simulink model "Inverted Pendulum stabilization_unstable_equilibrium"  (R2022b)
settings: Solver=VariableStepAuto  StartTime=0  StopTime=50  RelTol=1e-3
libraries: simulink x5, slpidlib x3
settings Model: Creator=Shaan Sapru  LastModifiedBy=Shaan Sapru
settings DataIOCC: SaveFormat=StructureWithTime
settings OptimizationCC: BlockReduction=off  BufferReuse=off
settings DebuggingCC: AlgebraicLoopMsg=none
settings ExplorerConfigSet: SimMechanicsOpenEditorOnUpdate=off

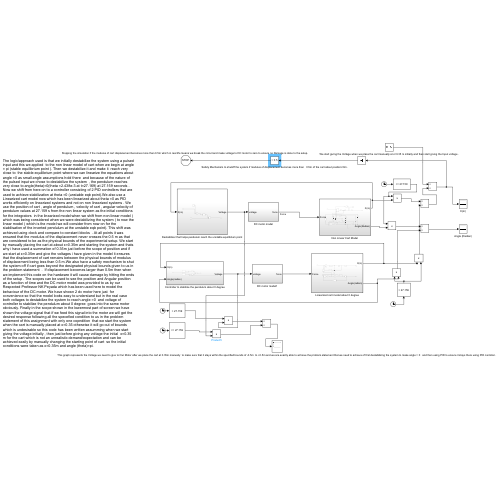
[thumbnail: Simulink's stored preview of the top-level diagram]
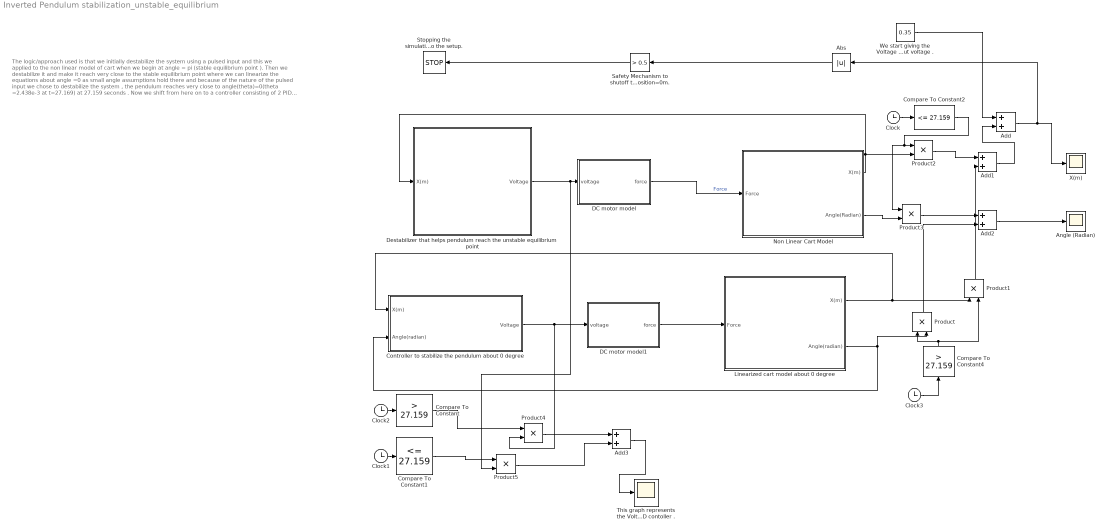
== system Inverted Pendulum stabilization_unstable_equilibrium ==
  note: The logic/approach used is that we initially destabilize the system using a pulsed input and this we applied to the non linear model of cart when we begin at angle = pi (stable equilibrium point ). Then we destabilize it and make it reach very close to the stable equilibrium point where we can linearize the equations about angle =0 as small angle assumptions hold there and because of the nature of the pulsed input we chose to destabilize the system , the pendulum reaches very close to angle(theta)=0(theta =2.438e-3 at t=27.169) at 27.159 seconds . Now we shift from here on to a controller consisting of 2 PID controllers that are used to achieve stabilization at theta =0 (unstable eqb point).We also use a Linearized cart model now which has been linearized about theta =0 as PID works efficiently on linearized systems and not on non linearized systems . We use the position of cart , angle of pendulum , velocity of cart , angular velocity of pendulum values at 27.159 s from the non linear system as the initial conditions for the integrators in the linearized model when we shift from non linear model ( which was being considered when we were destabilizing the system ) to now the linear model ( which is the model we will consider from now on for the stabilisation of the inverted pendulum at the unstable eqb point). This shift was achieved using clock and compare to constant blocks . At all points it was ensured that the modulus of the displacement never crosses the 0.5 m as that are considered to be as the physical bounds of the experimental setup. We start by manually placing the cart at about x=0.35m and starting the system and thats why i have used a summation of 0.35m just before the scope of position and if we start at x=0.35m and give the voltages i have given in the model it ensures that the displacement of cart remains between the physical bounds of modulus of displacement being less than 0.5 m.We also have a safety mechanism to shut the system off if cart goes beyond the designated physical bounds given to us in the problem statement . If displacement becomes larger than 0.5m then when we implement this code on the hardware it will cause damage by hitting the ends of the setup . The scopes can be used to see the position and Angular position as a function of time and the DC motor model was provided to us by our Respected Professor NK Peyada which has been used here to model the behaviour of the DC motor. We have shown 2 dc motor here just for convenience so that the model looks easy to understand but in the real case both voltages to destabilize the system to reach angle =0 and voltage of controller to stabilize the pendulum about 0 degree goes into the same motor obviously. Finally in the scope shown in the lowermost part of screen we have shown the voltage signal that if we feed this signal into the motor we will get the desired response following all the specefied condition to us in the problem statement of this assignment with only one copndition that we start the system when the cart is manually placed at x=0.35 otherwise it will go out of bounds which is undesirable so this code has been written assumming when we start giving the voltage initially , then just before giving any voltage the initial x=0.35 m for the cart which is not an unrealistic demand/expectation and can be achieved easily by manually changing the starting point of cart so the initial conditions were taken as x=0.35m and angle (theta)=pi.
  Abs : Abs  SaturateOnIntegerOverflow=off
  Add{,1..3} (4 alike) : Sum
  Angle (Radian) : Scope
  Clock{,1..3} (4 alike) : Clock
  Compare To Constant : simulink/Logic and Bit Operations/Compare To Constant  relop=>  const=27.159  OutDataTypeStr=boolean
  Compare To Constant1 : simulink/Logic and Bit Operations/Compare To Constant  relop=<=  const=27.159  OutDataTypeStr=boolean
  Compare To Constant2 : simulink/Logic and Bit Operations/Compare To Constant  relop=<=  const=27.159  OutDataTypeStr=boolean
  Compare To Constant4 : simulink/Logic and Bit Operations/Compare To Constant  relop=>  const=27.159  OutDataTypeStr=boolean
  Controller to stabilize the pendulum about 0 degree : Subsystem
  DC motor model : Subsystem
  DC motor model1 : Subsystem
  Destabilizer that helps pendulum reach the unstable equilibrium point : Subsystem
  Linearized cart model about 0 degree : Subsystem
  "Non Linear Cart Model " : Subsystem
  Product{,1..5} (6 alike) : Product
  Safety Mechanism to shutoff the system if modulus of displacement becomes more than   0.5m of the cart about position=0m. : simulink/Logic and Bit Operations/Compare To Constant  relop=>  const=0.5  OutDataTypeStr=boolean
  "Stopping the simulation if the modulus of cart displacement becomes more than 0.5m which in real life means we break the circuit and make voltage to DC motor to zero to ensure no Damage is done to the setup.  " : Stop
  "This graph represents the Voltage we need to give to Our Motor after we place the cart at 0.35m manually  to make sure that it stays within the specified bounds of -0.5m  to +0.5m and we are exactly able to achieve the problem statement that we need to achieve of first destabilizing the system to make angle = 0   and then using PID to ensure it stays there using PID contoller . " : Scope
  We start giving the Voltage when we place the cart manually at x=0.35 m initially and then start giving the Input voltage . : Constant  Value=0.35
  X(m) : Scope
  wires:
  DC motor model/1(force) -> "Non Linear Cart Model "/1(Force)  "Force"
  "Non Linear Cart Model "/1(X(m)) -> Product2/2, Destabilizer that helps pendulum reach the unstable equilibrium point/1(X(m))
  Destabilizer that helps pendulum reach the unstable equilibrium point/1(Voltage) -> Product5/2, DC motor model/1(voltage)
  DC motor model1/1(force) -> Linearized cart model about 0 degree/1(Force)
  Linearized cart model about 0 degree/1(X(m)) -> Controller to stabilize the pendulum about 0 degree/1(X(m)), Product1/1
  Linearized cart model about 0 degree/2(Angle(radian)) -> Controller to stabilize the pendulum about 0 degree/2(Angle(radian)), Product/2
  Add2/1 -> Angle (Radian)/1
  Add1/1 -> Add/2
  Product/1 -> Add2/2
  Product1/1 -> Add1/2
  Controller to stabilize the pendulum about 0 degree/1(Voltage) -> Product4/2, DC motor model1/1(voltage)
  Clock3/1 -> Compare To Constant4/1
  Compare To Constant4/1 -> Product/1, Product1/2
  Clock/1 -> Compare To Constant2/1
  Compare To Constant2/1 -> Product3/1, Product2/1
  Product2/1 -> Add1/1
  "Non Linear Cart Model "/2(Angle(Radian)) -> Product3/2
  Product3/1 -> Add2/1
  Safety Mechanism to shutoff the system if modulus of displacement becomes more than   0.5m of the cart about position=0m./1 -> "Stopping the simulation if the modulus of cart displacement becomes more than 0.5m which in real life means we break the circuit and make voltage to DC motor to zero to ensure no Damage is done to the setup.  "/1
  Abs/1 -> Safety Mechanism to shutoff the system if modulus of displacement becomes more than   0.5m of the cart about position=0m./1
  We start giving the Voltage when we place the cart manually at x=0.35 m initially and then start giving the Input voltage ./1 -> Add/1
  Add/1 -> Abs/1, X(m)/1
  Add3/1 -> "This graph represents the Voltage we need to give to Our Motor after we place the cart at 0.35m manually  to make sure that it stays within the specified bounds of -0.5m  to +0.5m and we are exactly able to achieve the problem statement that we need to achieve of first destabilizing the system to make angle = 0   and then using PID to ensure it stays there using PID contoller . "/1
  Compare To Constant/1 -> Product4/1
  Compare To Constant1/1 -> Product5/1
  Clock1/1 -> Compare To Constant1/1
  Product5/1 -> Add3/2
  Clock2/1 -> Compare To Constant/1
  Product4/1 -> Add3/1

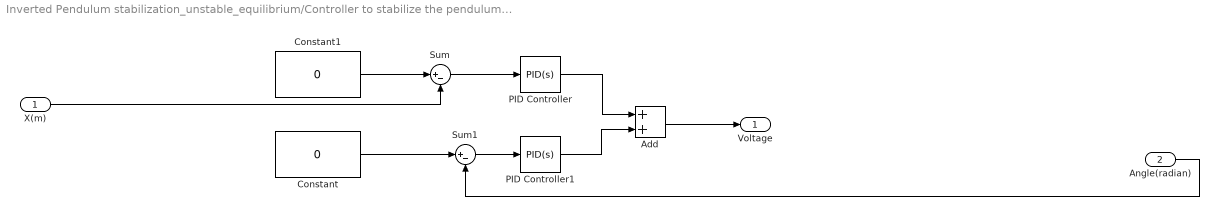
== system Inverted Pendulum stabilization_unstable_equilibrium/Controller to stabilize the pendulum about 0 degree ==
  X(m) : Inport
  Angle(radian) : Inport  Port=2
  Add : Sum
  Constant : Constant  Value=0
  Constant1 : Constant  Value=0
  PID Controller : slpidlib/PID Controller  Controller=PID  Form=Parallel  TimeDomain=Continuous-time  UseExternalTs=off  SampleTime=-1  IntegratorMethod=Forward Euler  FilterMethod=Forward Euler  ControllerParametersSource=internal  P=832.0243  I=93.876  UseKiTs=off  D=-197.943  N=4.2033  UseFilter=on  TunerSelectOption=Transfer Function Based (PID Tuner App)  InitialConditionSource=internal  InitialConditionForIntegrator=0  InitialConditionForFilter=0  DifferentiatorICPrevScaledInput=0  ExternalReset=none  TrackingMode=off  Kt=1  LimitOutput=off  SatLimitsSource=internal  UpperSaturationLimit=inf  LowerSaturationLimit=-inf  LinearizeAsGain=on  AntiWindupMode=none  Kb=1  LimitIntegrator=off  UpperIntegratorSaturationLimit=inf  LowerIntegratorSaturationLimit=-inf  POutMin=[]  POutMax=[]  IOutMin=[]  IOutMax=[]  DOutMin=[]  DOutMax=[]  NOutMin=[]  NOutMax=[]  SumOutMin=[]  SumOutMax=[]  SaturationOutMin=[]  SaturationOutMax=[]  PParamMin=[]  PParamMax=[]  IParamMin=[]  IParamMax=[]  DParamMin=[]  DParamMax=[]  NParamMin=[]  NParamMax=[]  KbParamMin=[]  KbParamMax=[]  KtParamMin=[]  KtParamMax=[]  KbOutMin=[]  KbOutMax=[]  KtOutMin=[]  KtOutMax=[]  IntegratorOutMin=[]  IntegratorOutMax=[]  FilterOutMin=[]  FilterOutMax=[]  SumI1OutMin=[]  SumI1OutMax=[]  SumI2OutMin=[]  SumI2OutMax=[]  SumI3OutMin=[]  SumI3OutMax=[]  SumI4OutMin=[]  SumI4OutMax=[]  SumDOutMin=[]  SumDOutMax=[]  DifferentiatorOutMin=[]  DifferentiatorOutMax=[]  FilterDiffOutCoefMin=[]  FilterDiffOutCoefMax=[]  ReciprocalOutMin=[]  ReciprocalOutMax=[]  SumDenOutMin=[]  SumDenOutMax=[]  SumNumOutMin=[]  SumNumOutMax=[]  DivideOutMin=[]  DivideOutMax=[]  UdiffTsProdOutMin=[]  UdiffTsProdOutMax=[]  NTsProdOutMin=[]  NTsProdOutMax=[]  UintegralTsProdOutMin=[]  UintegralTsProdOutMax=[]  UngainTsProdOutMin=[]  UngainTsProdOutMax=[]  ClampingZeroOutDataTypeStr=Inherit: Inherit via back propagation  ClampingZeroOutMin=[]  ClampingZeroOutMax=[]  FilterDenConstantOutDataTypeStr=Inherit: Inherit via back propagation  FilterDenConstantOutMin=[]  FilterDenConstantOutMax=[]  PCopyOutDataTypeStr=Inherit: Inherit via back propagation  PCopyOutMin=[]  PCopyOutMax=[]  NCopyOutDataTypeStr=Inherit: Inherit via back propagation  NCopyOutMin=[]  NCopyOutMax=[]  IntegratorContinuousStateAttributes=''  IntegratorStateMustResolveToSignalObject=off  IntegratorRTWStateStorageClass=Auto  FilterContinuousStateAttributes=''  FilterStateMustResolveToSignalObject=off  FilterRTWStateStorageClass=Auto  ParallelPVariant=InternalParameters  IdealPVariant=Disabled  IVariant=InternalParameters  DVariant=InternalParameters  IntegratorVariant=Continuous  SatVariant=Disabled  AWVariant=Passthrough  PCopyVariant=Disabled  TRVariant=Disabled  FdbkBlocksVariant=Forward  IdealPFdbkVariant=Disabled  SatFdbkVariant=Disabled  DerivativeFilterVariant=ContFilter  NVariant=InternalParameters  NCopyVariant=Disabled  FilterICVariant=InternalICsFilter  IntegratorICVariant=InternalICs  ExternalResetVariant=Disabled  TRSumVariant=Passthrough  SumFdbkVariant=Disabled  SumVariant=Sum_PID  TsampFilterVariant=InternalTs  TsampNgainVariant=Passthrough  TsampIntegralVariant=Passthrough  ExternalSaturationOutDataTypeStr=Inherit: Same as second input
  PID Controller1 : slpidlib/PID Controller  Controller=PID  Form=Parallel  TimeDomain=Continuous-time  UseExternalTs=off  SampleTime=-1  IntegratorMethod=Forward Euler  FilterMethod=Forward Euler  ControllerParametersSource=internal  P=2215.083  I=8077.564  UseKiTs=off  D=0  N=100  UseFilter=on  TunerSelectOption=Transfer Function Based (PID Tuner App)  InitialConditionSource=internal  InitialConditionForIntegrator=0  InitialConditionForFilter=0  DifferentiatorICPrevScaledInput=0  ExternalReset=none  TrackingMode=off  Kt=1  LimitOutput=off  SatLimitsSource=internal  UpperSaturationLimit=inf  LowerSaturationLimit=-inf  LinearizeAsGain=on  AntiWindupMode=none  Kb=1  LimitIntegrator=off  UpperIntegratorSaturationLimit=inf  LowerIntegratorSaturationLimit=-inf  POutMin=[]  POutMax=[]  IOutMin=[]  IOutMax=[]  DOutMin=[]  DOutMax=[]  NOutMin=[]  NOutMax=[]  SumOutMin=[]  SumOutMax=[]  SaturationOutMin=[]  SaturationOutMax=[]  PParamMin=[]  PParamMax=[]  IParamMin=[]  IParamMax=[]  DParamMin=[]  DParamMax=[]  NParamMin=[]  NParamMax=[]  KbParamMin=[]  KbParamMax=[]  KtParamMin=[]  KtParamMax=[]  KbOutMin=[]  KbOutMax=[]  KtOutMin=[]  KtOutMax=[]  IntegratorOutMin=[]  IntegratorOutMax=[]  FilterOutMin=[]  FilterOutMax=[]  SumI1OutMin=[]  SumI1OutMax=[]  SumI2OutMin=[]  SumI2OutMax=[]  SumI3OutMin=[]  SumI3OutMax=[]  SumI4OutMin=[]  SumI4OutMax=[]  SumDOutMin=[]  SumDOutMax=[]  DifferentiatorOutMin=[]  DifferentiatorOutMax=[]  FilterDiffOutCoefMin=[]  FilterDiffOutCoefMax=[]  ReciprocalOutMin=[]  ReciprocalOutMax=[]  SumDenOutMin=[]  SumDenOutMax=[]  SumNumOutMin=[]  SumNumOutMax=[]  DivideOutMin=[]  DivideOutMax=[]  UdiffTsProdOutMin=[]  UdiffTsProdOutMax=[]  NTsProdOutMin=[]  NTsProdOutMax=[]  UintegralTsProdOutMin=[]  UintegralTsProdOutMax=[]  UngainTsProdOutMin=[]  UngainTsProdOutMax=[]  ClampingZeroOutDataTypeStr=Inherit: Inherit via back propagation  ClampingZeroOutMin=[]  ClampingZeroOutMax=[]  FilterDenConstantOutDataTypeStr=Inherit: Inherit via back propagation  FilterDenConstantOutMin=[]  FilterDenConstantOutMax=[]  PCopyOutDataTypeStr=Inherit: Inherit via back propagation  PCopyOutMin=[]  PCopyOutMax=[]  NCopyOutDataTypeStr=Inherit: Inherit via back propagation  NCopyOutMin=[]  NCopyOutMax=[]  IntegratorContinuousStateAttributes=''  IntegratorStateMustResolveToSignalObject=off  IntegratorRTWStateStorageClass=Auto  FilterContinuousStateAttributes=''  FilterStateMustResolveToSignalObject=off  FilterRTWStateStorageClass=Auto  ParallelPVariant=InternalParameters  IdealPVariant=Disabled  IVariant=InternalParameters  DVariant=InternalParameters  IntegratorVariant=Continuous  SatVariant=Disabled  AWVariant=Passthrough  PCopyVariant=Disabled  TRVariant=Disabled  FdbkBlocksVariant=Forward  IdealPFdbkVariant=Disabled  SatFdbkVariant=Disabled  DerivativeFilterVariant=ContFilter  NVariant=InternalParameters  NCopyVariant=Disabled  FilterICVariant=InternalICsFilter  IntegratorICVariant=InternalICs  ExternalResetVariant=Disabled  TRSumVariant=Passthrough  SumFdbkVariant=Disabled  SumVariant=Sum_PID  TsampFilterVariant=InternalTs  TsampNgainVariant=Passthrough  TsampIntegralVariant=Passthrough  ExternalSaturationOutDataTypeStr=Inherit: Same as second input
  Sum : Sum  Inputs=|+-
  Sum1 : Sum  Inputs=|+-
  Voltage : Outport
  wires:
  Constant1/1 -> Sum/1
  PID Controller1/1 -> Add/2
  Add/1 -> Voltage/1
  Constant/1 -> Sum1/1
  PID Controller/1 -> Add/1
  Sum1/1 -> PID Controller1/1
  X(m)/1 -> Sum/2
  Sum/1 -> PID Controller/1
  Angle(radian)/1 -> Sum1/2

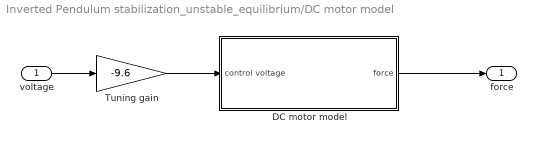
== system Inverted Pendulum stabilization_unstable_equilibrium/DC motor model ==
  voltage : Inport
  DC motor model : Subsystem  mask{J=0.0000140, Kt=0.05, Kb=0.05, d=0.000001, R=2.5, L=0.0025}
      mask prompts: J "Moment of inertia"; Kt "Torque constant"; Kb "Electromotive force constant"; d "Linear approximation of viscous friction"; R "Electrical circuit resistance"; L "Electrical circuit inductance"
      mask Display: disp('DC motor')
  Tuning gain : Gain  Gain=-9.6
  force : Outport
  wires:
  Tuning gain/1 -> DC motor model/1(control voltage)
  voltage/1 -> Tuning gain/1
  DC motor model/1(force) -> force/1

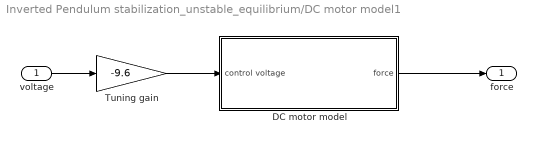
== system Inverted Pendulum stabilization_unstable_equilibrium/DC motor model1 ==
  voltage : Inport
  DC motor model : Subsystem  mask{J=0.0000140, Kt=0.05, Kb=0.05, d=0.000001, R=2.5, L=0.0025}
      mask prompts: J "Moment of inertia"; Kt "Torque constant"; Kb "Electromotive force constant"; d "Linear approximation of viscous friction"; R "Electrical circuit resistance"; L "Electrical circuit inductance"
      mask Display: disp('DC motor')
  Tuning gain : Gain  Gain=-9.6
  force : Outport
  wires:
  Tuning gain/1 -> DC motor model/1(control voltage)
  voltage/1 -> Tuning gain/1
  DC motor model/1(force) -> force/1

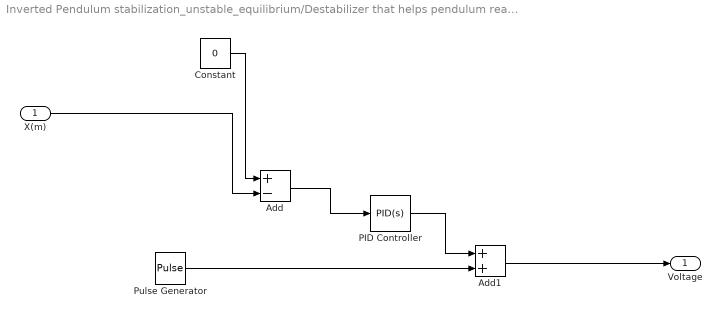
== system Inverted Pendulum stabilization_unstable_equilibrium/Destabilizer that helps pendulum reach the unstable equilibrium point ==
  X(m) : Inport
  Add : Sum  Inputs=+-
  Add1 : Sum
  Constant : Constant  Value=0
  PID Controller : slpidlib/PID Controller  Controller=PID  Form=Parallel  TimeDomain=Continuous-time  UseExternalTs=off  SampleTime=-1  IntegratorMethod=Forward Euler  FilterMethod=Forward Euler  ControllerParametersSource=internal  P=-0.689804794145449  I=-0.0287985752446261  UseKiTs=off  D=-0.351556934511218  N=2.44257175027819  UseFilter=on  TunerSelectOption=Transfer Function Based (PID Tuner App)  InitialConditionSource=internal  InitialConditionForIntegrator=0  InitialConditionForFilter=0  DifferentiatorICPrevScaledInput=0  ExternalReset=none  TrackingMode=off  Kt=1  LimitOutput=off  SatLimitsSource=internal  UpperSaturationLimit=inf  LowerSaturationLimit=-inf  LinearizeAsGain=on  AntiWindupMode=none  Kb=1  LimitIntegrator=off  UpperIntegratorSaturationLimit=inf  LowerIntegratorSaturationLimit=-inf  POutMin=[]  POutMax=[]  IOutMin=[]  IOutMax=[]  DOutMin=[]  DOutMax=[]  NOutMin=[]  NOutMax=[]  SumOutMin=[]  SumOutMax=[]  SaturationOutMin=[]  SaturationOutMax=[]  PParamMin=[]  PParamMax=[]  IParamMin=[]  IParamMax=[]  DParamMin=[]  DParamMax=[]  NParamMin=[]  NParamMax=[]  KbParamMin=[]  KbParamMax=[]  KtParamMin=[]  KtParamMax=[]  KbOutMin=[]  KbOutMax=[]  KtOutMin=[]  KtOutMax=[]  IntegratorOutMin=[]  IntegratorOutMax=[]  FilterOutMin=[]  FilterOutMax=[]  SumI1OutMin=[]  SumI1OutMax=[]  SumI2OutMin=[]  SumI2OutMax=[]  SumI3OutMin=[]  SumI3OutMax=[]  SumI4OutMin=[]  SumI4OutMax=[]  SumDOutMin=[]  SumDOutMax=[]  DifferentiatorOutMin=[]  DifferentiatorOutMax=[]  FilterDiffOutCoefMin=[]  FilterDiffOutCoefMax=[]  ReciprocalOutMin=[]  ReciprocalOutMax=[]  SumDenOutMin=[]  SumDenOutMax=[]  SumNumOutMin=[]  SumNumOutMax=[]  DivideOutMin=[]  DivideOutMax=[]  UdiffTsProdOutMin=[]  UdiffTsProdOutMax=[]  NTsProdOutMin=[]  NTsProdOutMax=[]  UintegralTsProdOutMin=[]  UintegralTsProdOutMax=[]  UngainTsProdOutMin=[]  UngainTsProdOutMax=[]  ClampingZeroOutDataTypeStr=Inherit: Inherit via back propagation  ClampingZeroOutMin=[]  ClampingZeroOutMax=[]  FilterDenConstantOutDataTypeStr=Inherit: Inherit via back propagation  FilterDenConstantOutMin=[]  FilterDenConstantOutMax=[]  PCopyOutDataTypeStr=Inherit: Inherit via back propagation  PCopyOutMin=[]  PCopyOutMax=[]  NCopyOutDataTypeStr=Inherit: Inherit via back propagation  NCopyOutMin=[]  NCopyOutMax=[]  IntegratorContinuousStateAttributes=''  IntegratorStateMustResolveToSignalObject=off  IntegratorRTWStateStorageClass=Auto  FilterContinuousStateAttributes=''  FilterStateMustResolveToSignalObject=off  FilterRTWStateStorageClass=Auto  ParallelPVariant=InternalParameters  IdealPVariant=Disabled  IVariant=InternalParameters  DVariant=InternalParameters  IntegratorVariant=Continuous  SatVariant=Disabled  AWVariant=Passthrough  PCopyVariant=Disabled  TRVariant=Disabled  FdbkBlocksVariant=Forward  IdealPFdbkVariant=Disabled  SatFdbkVariant=Disabled  DerivativeFilterVariant=ContFilter  NVariant=InternalParameters  NCopyVariant=Disabled  FilterICVariant=InternalICsFilter  IntegratorICVariant=InternalICs  ExternalResetVariant=Disabled  TRSumVariant=Passthrough  SumFdbkVariant=Disabled  SumVariant=Sum_PID  TsampFilterVariant=InternalTs  TsampNgainVariant=Passthrough  TsampIntegralVariant=Passthrough  ExternalSaturationOutDataTypeStr=Inherit: Same as second input
  Pulse Generator : DiscretePulseGenerator  PulseType=Time based  Amplitude=23.87  Period=2.683*2
  Voltage : Outport
  wires:
  Add/1 -> PID Controller/1
  Pulse Generator/1 -> Add1/2
  PID Controller/1 -> Add1/1
  Constant/1 -> Add/1
  X(m)/1 -> Add/2
  Add1/1 -> Voltage/1

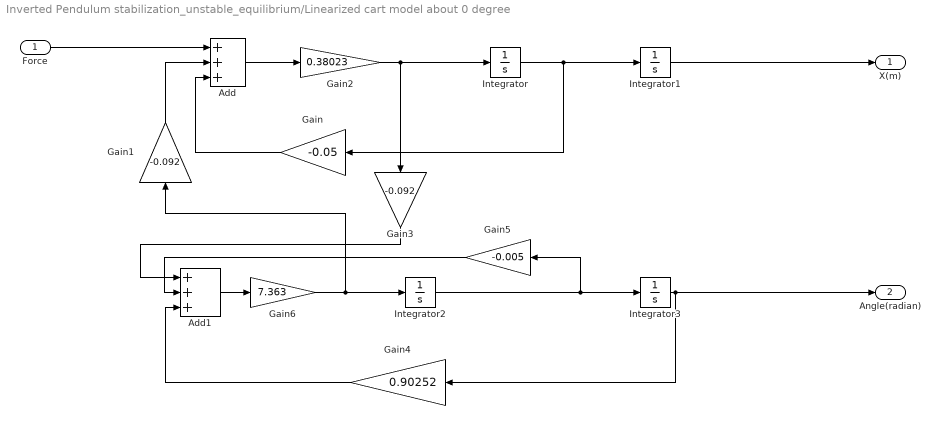
== system Inverted Pendulum stabilization_unstable_equilibrium/Linearized cart model about 0 degree ==
  Force : Inport
  Add : Sum  Inputs=+++
  Add1 : Sum  Inputs=+++
  Gain : Gain  Gain=-0.05
  Gain1 : Gain  Gain=-0.092
  Gain2 : Gain  Gain=0.38023
  Gain3 : Gain  Gain=-0.092
  Gain4 : Gain  Gain=0.90252
  Gain5 : Gain  Gain=-0.005
  Gain6 : Gain  Gain=7.363
  Integrator : Integrator  InitialCondition=0.655
  Integrator1 : Integrator  InitialCondition=-0.4909
  Integrator2 : Integrator  InitialCondition=-6.178
  Integrator3 : Integrator  InitialCondition=2.438e-3
  X(m) : Outport
  Angle(radian) : Outport  Port=2
  wires:
  Gain1/1 -> Add/2
  Integrator2/1 -> Gain5/1, Integrator3/1
  Integrator3/1 -> Gain4/1, Angle(radian)/1
  Gain2/1 -> Gain3/1, Integrator/1
  Add1/1 -> Gain6/1
  Gain4/1 -> Add1/3
  Gain/1 -> Add/3
  Integrator1/1 -> X(m)/1
  Integrator/1 -> Gain/1, Integrator1/1
  Force/1 -> Add/1
  Add/1 -> Gain2/1
  Gain3/1 -> Add1/1
  Gain5/1 -> Add1/2
  Gain6/1 -> Integrator2/1, Gain1/1

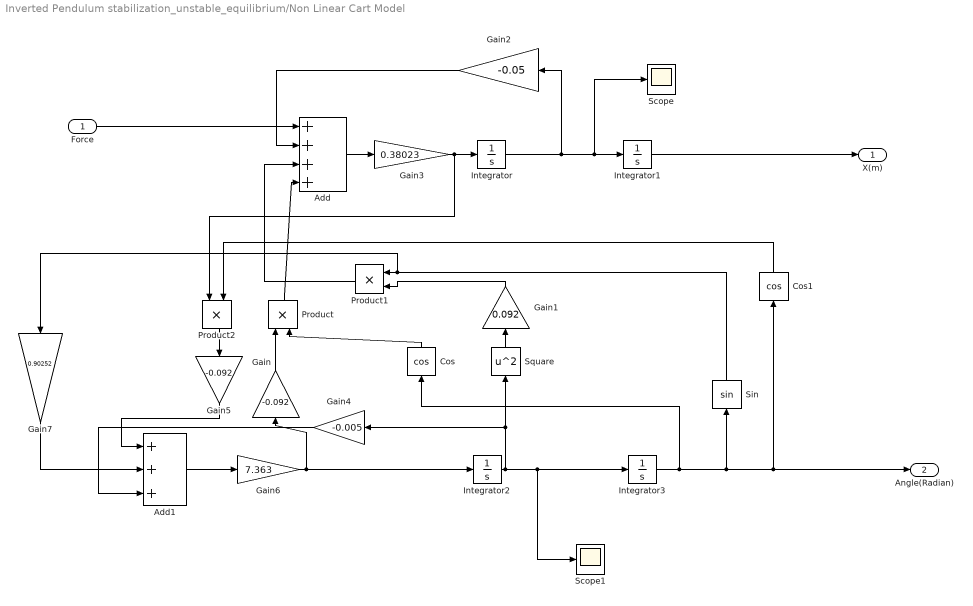
== system Inverted Pendulum stabilization_unstable_equilibrium/Non Linear Cart Model  ==
  Force : Inport
  Add : Sum  Inputs=++++
  Add1 : Sum  Inputs=+++
  Cos : Trigonometry  Operator=cos
  Cos1 : Trigonometry  Operator=cos
  Gain : Gain  Gain=-0.092
  Gain1 : Gain  Gain=0.092
  Gain2 : Gain  Gain=-0.05
  Gain3 : Gain  Gain=0.38023
  Gain4 : Gain  Gain=-0.005
  Gain5 : Gain  Gain=-0.092
  Gain6 : Gain  Gain=7.363
  Gain7 : Gain  Gain=0.90252
  Integrator : Integrator
  Integrator1 : Integrator
  Integrator2 : Integrator
  Integrator3 : Integrator  InitialCondition=pi
  Product : Product
  Product1 : Product
  Product2 : Product
  Scope : Scope
  Scope1 : Scope
  Sin : Trigonometry
  Square : Math  Operator=square
  X(m) : Outport
  Angle(Radian) : Outport  Port=2
  wires:
  Integrator3/1 -> Cos/1, Sin/1, Cos1/1, Angle(Radian)/1
  Integrator2/1 -> Square/1, Gain4/1, Scope1/1, Integrator3/1
  Integrator/1 -> Scope/1, Integrator1/1, Gain2/1
  Integrator1/1 -> X(m)/1
  Force/1 -> Add/1
  Add1/1 -> Gain6/1
  Cos/1 -> Product/2
  Gain/1 -> Product/1
  Product/1 -> Add/4
  Square/1 -> Gain1/1
  Gain1/1 -> Product1/2
  Product1/1 -> Add/3
  Sin/1 -> Gain7/1, Product1/1
  Gain2/1 -> Add/2
  Add/1 -> Gain3/1
  Gain3/1 -> Product2/1, Integrator/1
  Gain6/1 -> Gain/1, Integrator2/1
  Gain4/1 -> Add1/3
  Cos1/1 -> Product2/2
  Product2/1 -> Gain5/1
  Gain5/1 -> Add1/1
  Gain7/1 -> Add1/2

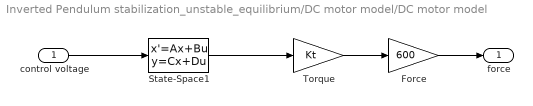
== system Inverted Pendulum stabilization_unstable_equilibrium/DC motor model/DC motor model ==
  control voltage : Inport
  Force : Gain  Gain=600
  State-Space1 : StateSpace  A=[-d/J Kt/J;-Kb/L -R/L]  B=[0; 1/L]  C=[0 1]  D=0  InitialCondition=0
  Torque : Gain  Gain=Kt
  force : Outport
  wires:
  control voltage/1 -> State-Space1/1
  State-Space1/1 -> Torque/1
  Torque/1 -> Force/1
  Force/1 -> force/1

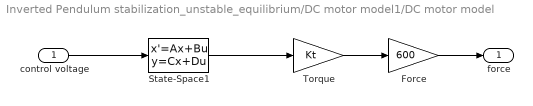
== system Inverted Pendulum stabilization_unstable_equilibrium/DC motor model1/DC motor model ==
  control voltage : Inport
  Force : Gain  Gain=600
  State-Space1 : StateSpace  A=[-d/J Kt/J;-Kb/L -R/L]  B=[0; 1/L]  C=[0 1]  D=0  InitialCondition=0
  Torque : Gain  Gain=Kt
  force : Outport
  wires:
  control voltage/1 -> State-Space1/1
  State-Space1/1 -> Torque/1
  Torque/1 -> Force/1
  Force/1 -> force/1
